simulink model "test"  (R2019a)
settings: Solver=FixedStepAuto  StartTime=0.0  StopTime=tf  FixedStep=ts  RelTol=1e-3
values from neighbouring files (symbols this model uses):
  k_d = 8    [initial.m]
  k_p = 25    [initial.m]
  x0 = [-0.1 0.1]    [initial.m]
settings Model: Creator=AMIN  LastModifiedBy=AMIN
settings DataIOCC: SaveFormat=Array  ReturnWorkspaceOutputs=off

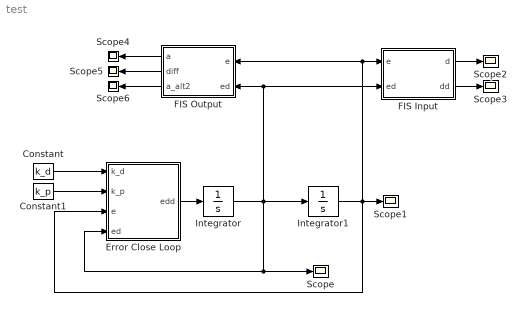
== system test ==
  Constant : Constant  Value=k_d
  Constant1 : Constant  Value=k_p
  Error Close Loop : MATLAB Function  TreatAsAtomicUnit=on
  FIS Input : MATLAB Function  TreatAsAtomicUnit=on
  FIS Output : MATLAB Function  TreatAsAtomicUnit=on
  Integrator : Integrator
  Integrator1 : Integrator  InitialCondition=x0
  Scope{,1..6} (7 alike) : Scope
  wires:
  Error Close Loop/1(edd) -> Integrator/1
  Integrator1/1 -> FIS Input/1(e), FIS Output/1(e), Scope1/1, Error Close Loop/3(e)
  Constant/1 -> Error Close Loop/1(k_d)
  Constant1/1 -> Error Close Loop/2(k_p)
  Integrator/1 -> FIS Input/2(ed), FIS Output/2(ed), Integrator1/1, Scope/1, Error Close Loop/4(ed)
  FIS Input/1(d) -> Scope2/1
  FIS Input/2(dd) -> Scope3/1
  FIS Output/1(a) -> Scope4/1
  FIS Output/3(a_alt2) -> Scope6/1
  FIS Output/2(diff) -> Scope5/1

== matlab function test/FIS Input ==
  data: e input; ed input; d output; dd output
function [d,dd] = fcn(e,ed)
d = norm(e);
dd = norm(ed)*sign(sign(ed(1))+sign(ed(2))-1);
end

== matlab function test/Error Close Loop ==
  data: k_d input; k_p input; edd output; e input; ed input
function edd = fcn(k_d,k_p,e,ed)
edd = - k_d*ed - k_p*e;
end

== matlab function test/FIS Output ==
  data: e input; ed input; a output; diff output; a_alt2 output
function [a,diff,a_alt2] = fcn(e,ed)
%% method 1
 a = norm(ed);
%% method 2
 d = norm(e);
 a1 = ed(1)*d/e(1);
 a2 = ed(1)*d/e(2);
 a_alt2 = norm([a1 a2]);
 diff = a_alt2 - a;
end
